simulink library "pathFollowingControllerExpStateMachine_cl"  (R2020a)
settings: Solver=VariableStepAuto  StartTime=0.0  StopTime=10.0  RelTol=1e-3
undefined symbols (not defined in the file or in its folder): env, FLIGHTCONTROLLER, fltCtrl, initializeBussesFromBlock, vhcl
libraries: simulink x6, filteredPIDController_ul x3, velocityAngle_ul x3, eulAng2RotMat_ul x2, stopwatch_ul x1, dspsigops x1, courseFollowExp_cl x1, ctrlAllocMatrixExp_cl x1, angleBtw2Vecs_ul x1, vrlib x1, alphaBeta_ul x1, gnd2TanRotation_ul x1
settings Model: Creator=jldanie5  LastModifiedBy=jcreed2
settings DataIOCC: ReturnWorkspaceOutputs=off
settings DebuggingCC: ArithmeticOperatorsInVariantConditions=warning
settings SFSimCC: CustomCodeUndefinedFunction=UseInterfaceOnly

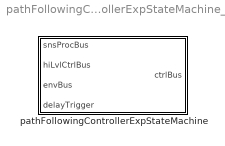
== system pathFollowingControllerExpStateMachine_cl ==
  pathFollowingControllerExpStateMachine : Subsystem  LoadFcn=initializeBussesFromBlock(gcb)  InitFcn=initializeBussesFromBlock(gcb)  StartFcn=initializeBussesFromBlock(gcb)  VariantControl=strcmpi(FLIGHTCONTROLLER,'pathFollowingControllerMantaBandLin')  mask{initPosForInitSStar=vhcl.initPosVecGnd.Value, fluidDensity=env.water.density.Value, pathCtrl=fltCtrl, aeroStruct=vhcl.struct('OCT.aeroSurf'), thrAttach=vhcl.rBridle_LE.Value, vhcl=vhcl}
      mask prompts: initPosForInitSStar "Initial Position"; fluidDensity "Fluid Density"; pathCtrl "Controller"; aeroStruct "Aerodynamic Structure"; thrAttach "Tether Attach Point"; vhcl "Vehicle"
      settings: MinAlgLoopOccurrences=on
      mask DialogControl Container3 Prompt: courseFollow Params
      mask DialogControl Container4 Prompt: setpointToOutput Params

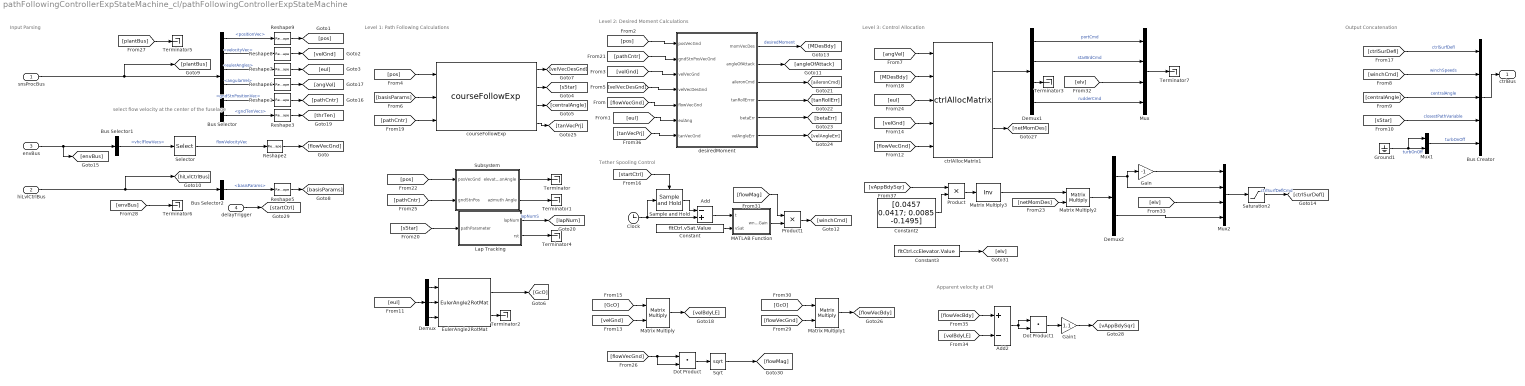
== system pathFollowingControllerExpStateMachine_cl/pathFollowingControllerExpStateMachine ==
  note: select flow velocity at the center of the fuselage
  note: Level 3: Control Allocation
  note: Output Concatenation
  note: Tether Spooling Control
  note: Level 2: Desired Moment Calculations
  note: Level 1: Path Following Calculations
  note: Input Parsing
  note: Apparent velocity at CM
  snsProcBus : Inport  OutDataTypeStr=Bus: sensorsProcessingBus
  hiLvlCtrlBus : Inport  Port=2  OutDataTypeStr=Bus: hiLvlCtrlBus
  envBus : Inport  Port=3  OutDataTypeStr=Bus: envBus
  delayTrigger : Inport  Port=4
  Add : Sum  Inputs=-+
  Add2 : Sum  Inputs=+-
  Bus Creator : BusCreator  Inputs=5  OutDataTypeStr=Bus: fltCtrlBus
      settings: InheritFromInputs=off
  Bus Selector : BusSelector  OutputSignals=positionVec,velocityVec,eulerAngles,angularVel,gndStnPositionVec,gndTenVecs
  Bus Selector1 : BusSelector  OutputSignals=vhclFlowVecs
  Bus Selector2 : BusSelector  OutputSignals=basisParams
  Clock : Clock
  Constant : Constant  Value=fltCtrl.vSat.Value
  Constant2 : Constant  Value=[0.0457 0.0417; 0.0085 -0.1495]
  Constant3 : Constant  Value=fltCtrl.ccElevator.Value
  Demux : Demux  Outputs=3
  Demux1 : Demux
  Demux2 : Demux  Outputs=2
  Dot Product : DotProduct  InputSameDT=on  OutDataTypeStr=Inherit: Inherit via internal rule
  Dot Product1 : DotProduct  InputSameDT=on  OutDataTypeStr=Inherit: Inherit via internal rule
  EulerAngle2RotMat : eulAng2RotMat_ul/EulerAngle2RotMat  SystemSampleTime=-1  Latency=0  AutoFrameSizeCalculation=off
  Gain : Gain  Gain=-1
  Gain1 : Gain  Gain=1.1
  Ground1 : Ground
  Lap Tracking : Subsystem
  MATLAB Function : MATLAB Function  TreatAsAtomicUnit=on
  Matrix Multiply : Product  Multiplication=Matrix(*)
  Matrix Multiply1 : Product  Multiplication=Matrix(*)
  Matrix Multiply2 : Product  Multiplication=Matrix(*)
  Matrix Multiply3 : Product  Inputs=/  Multiplication=Matrix(*)
  Mux : Mux
  Mux1 : Mux  Inputs=2
  Mux2 : Mux
  Product : Product
  Product1 : Product
  Reshape{1..3,5..9} (8 alike) : Reshape  OutputDimensionality=Column vector (2-D)
  Sample and Hold : dspsigops/Sample and Hold  trig=Rising edge  initCond=0  latchinput=off
  Saturation2 : Saturate  UpperLimit=pathCtrl.controlSigMax.upperLimit.Value  LowerLimit=pathCtrl.controlSigMax.lowerLimit.Value
  Selector : Selector  NumberOfDimensions=2  InputPortWidth=3  IndexOptions=Select all,Index vector (dialog)  Indices=[1 3],5  OutputSizes=1,1
  Sqrt : Sqrt  SaturateOnIntegerOverflow=on
  Subsystem : Subsystem
  Terminator{,1..7} (8 alike) : Terminator
  courseFollowExp : courseFollowExp_cl/courseFollowExp  SystemSampleTime=-1  Latency=0  AutoFrameSizeCalculation=off
  ctrlAllocMatrix1 : ctrlAllocMatrixExp_cl/ctrlAllocMatrix  aeroStruct=vhcl.struct('OCT.aeroSurf')  fluidDensity=fluidDensity
  desiredMoment : Subsystem
  ctrlBus : Outport  OutDataTypeStr=Bus: fltCtrlBus  VectorParamsAs1DForOutWhenUnconnected=off
  wires:
  Bus Selector/6 -> Reshape3/1  "<gndTenVecs>"
  Reshape3/1 -> [thrTen]
  courseFollowExp/1 -> [velVecDesGnd]
  snsProcBus/1 -> Bus Selector/1, [plantBus]
  Bus Selector/2 -> Reshape8/1  "<velocityVec>"
  Bus Selector/1 -> Reshape9/1  "<positionVec>"
  Bus Selector/3 -> Reshape7/1  "<eulerAngles>"
  [pos] -> courseFollowExp/1
  Bus Creator/1 -> ctrlBus/1
  [winchCmd] -> Bus Creator/2  "winchSpeeds"
  courseFollowExp/2 -> [sStar]
  hiLvlCtrlBus/1 -> [hiLvlCtrlBus], Bus Selector2/1
  [centralAngle] -> Bus Creator/3  "centralAngle"
  [sStar] -> Bus Creator/4  "closestPathVariable"
  courseFollowExp/3 -> [centralAngle]
  desiredMoment/1(momVecDes) -> [MDesBdy]  "desiredMoment"
  Bus Selector/4 -> Reshape6/1  "<angularVel>"
  [angVel] -> ctrlAllocMatrix1/1
  Demux1/3 -> Terminator3/1
  Demux1/1 -> Mux/1  "portCmd"
  Demux1/2 -> Mux/2  "starBrdCmd"
  ctrlAllocMatrix1/1 -> Demux1/1
  [ctrlSurDefl] -> Bus Creator/1  "ctrlSurfDefl"
  Bus Selector2/1 -> Reshape5/1  "<basisParams>"
  Reshape5/1 -> [basisParams]
  Saturation2/1 -> [ctrlSurDefl]  "ctrlSurfDeflCmd"
  Reshape2/1 -> [flowVecGnd]
  Reshape6/1 -> [angVel]
  Reshape7/1 -> [eul]
  Reshape8/1 -> [velGnd]
  Reshape9/1 -> [pos]
  Selector/1 -> Reshape2/1  "flowVelocityVec"
  envBus/1 -> [envBus], Bus Selector1/1
  Bus Selector1/1 -> Selector/1  "<vhclFlowVecs>"
  Reshape1/1 -> [pathCntr]
  Bus Selector/5 -> Reshape1/1  "<gndStnPositionVec>"
  [pathCntr] -> courseFollowExp/3
  [pos] -> desiredMoment/1(posVecGnd)
  [pathCntr] -> desiredMoment/2(gndStnPosVecGnd)
  [velGnd] -> desiredMoment/3(velVecGnd)
  [velVecDesGnd] -> desiredMoment/4(velVecDesGnd)
  [eul] -> desiredMoment/6(eulAng)
  [flowVecGnd] -> desiredMoment/5(flowVecGnd)
  [basisParams] -> courseFollowExp/2
  Demux1/4 -> Mux/4  "rudderCmd"
  Mux1/1 -> Bus Creator/5  "turbOnOff"
  [pos] -> Subsystem/1(posVecGnd)
  Subsystem/1(elevationAngle) -> Terminator/1
  Subsystem/2(azimuth Angle) -> Terminator1/1
  [elv] -> Mux/3
  desiredMoment/2(angleOfAttack) -> [angleOfAttack]
  [sStar] -> Lap Tracking/1(pathParameter)
  Lap Tracking/2(rst) -> Terminator4/1
  Lap Tracking/1(lapNum) -> [lapNum]  "lapNumS"
  [plantBus] -> Terminator5/1
  [envBus] -> Terminator6/1
  Constant/1 -> MATLAB Function/2(vSat)
  desiredMoment/3(aileronCmd) -> [aileronCmd]
  Mux/1 -> Terminator7/1
  desiredMoment/4(tanRollError) -> [tanRollErr]
  desiredMoment/5(betaErr) -> [betaErr]
  desiredMoment/6(velAngleErr) -> [velAngleErr]
  courseFollowExp/4 -> [tanVecPrj]
  [tanVecPrj] -> desiredMoment/7(tanVecGnd)
  [velGnd] -> ctrlAllocMatrix1/4
  [eul] -> ctrlAllocMatrix1/3
  [flowVecGnd] -> ctrlAllocMatrix1/5
  [MDesBdy] -> ctrlAllocMatrix1/2
  [pathCntr] -> Subsystem/2(gndStnPos)
  Ground1/1 -> Mux1/1, Mux1/2  "turbOnOff"
  [eul] -> Demux/1
  Demux/2 -> EulerAngle2RotMat/2
  Demux/1 -> EulerAngle2RotMat/1
  Demux/3 -> EulerAngle2RotMat/3
  EulerAngle2RotMat/2 -> Terminator2/1
  EulerAngle2RotMat/1 -> [GcO]
  [velGnd] -> Matrix Multiply/2
  [GcO] -> Matrix Multiply/1
  Matrix Multiply/1 -> [velBdyLE]
  Matrix Multiply1/1 -> [flowVecBdy]
  [GcO] -> Matrix Multiply1/1
  [flowVecGnd] -> Matrix Multiply1/2
  Constant2/1 -> Product/2
  Matrix Multiply2/1 -> Demux2/1
  Demux2/1 -> Mux2/2, Gain/1
  Gain/1 -> Mux2/1
  [elv] -> Mux2/3
  Demux2/2 -> Mux2/4
  Add2/1 -> Dot Product1/1, Dot Product1/2
  [flowVecBdy] -> Add2/1
  [velBdyLE] -> Add2/2
  Product/1 -> Matrix Multiply3/1
  Matrix Multiply3/1 -> Matrix Multiply2/1
  ctrlAllocMatrix1/2 -> [netMomDes]
  Dot Product1/1 -> Gain1/1
  [netMomDes] -> Matrix Multiply2/2
  [vAppBdySqr] -> Product/1
  Gain1/1 -> [vAppBdySqr]
  delayTrigger/1 -> [startCtrl]
  [startCtrl] -> Sample and Hold/Trigger
  Clock/1 -> Add/2, Sample and Hold/1
  Sample and Hold/1 -> Add/1
  Add/1 -> MATLAB Function/1(t)
  [flowVecGnd] -> Dot Product/2, Dot Product/1
  Dot Product/1 -> Sqrt/1
  Sqrt/1 -> [flowMag]
  MATLAB Function/1(wnchGain) -> Product1/2
  [flowMag] -> Product1/1
  Product1/1 -> [winchCmd]
  Constant3/1 -> [elv]
  Mux2/1 -> Saturation2/1

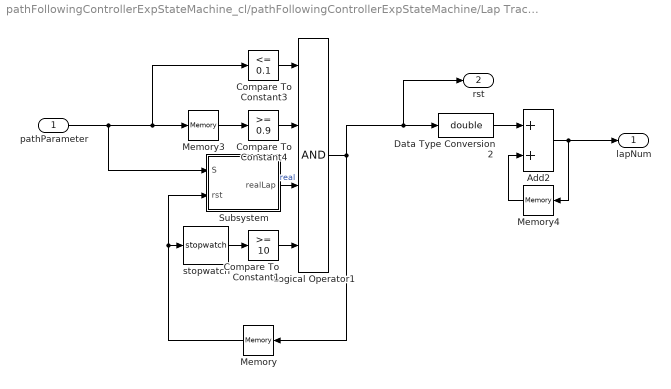
== system pathFollowingControllerExpStateMachine_cl/pathFollowingControllerExpStateMachine/Lap Tracking ==
  pathParameter : Inport
  Add2 : Sum
  Compare To Constant1 : simulink/Logic and Bit Operations/Compare To Constant  relop=>=  const=10  OutDataTypeStr=boolean
  Compare To Constant3 : simulink/Logic and Bit Operations/Compare To Constant  relop=<=  const=0.1  OutDataTypeStr=boolean
  Compare To Constant4 : simulink/Logic and Bit Operations/Compare To Constant  relop=>=  const=0.9  OutDataTypeStr=boolean
  Data Type Conversion2 : DataTypeConversion  OutDataTypeStr=double
  Logical Operator1 : Logic  Inputs=4  AllPortsSameDT=off  OutDataTypeStr=boolean
  Memory : Memory  InitialCondition=false
  Memory3 : Memory
  Memory4 : Memory
  Subsystem : Subsystem
  stopwatch : stopwatch_ul/stopwatch  SystemSampleTime=-1  Latency=0  AutoFrameSizeCalculation=off
  lapNum : Outport  VectorParamsAs1DForOutWhenUnconnected=off
  rst : Outport  Port=2  VectorParamsAs1DForOutWhenUnconnected=off
  wires:
  Compare To Constant3/1 -> Logical Operator1/1
  Memory3/1 -> Compare To Constant4/1
  Data Type Conversion2/1 -> Add2/1
  Logical Operator1/1 -> rst/1, Data Type Conversion2/1, Memory/1
  Memory4/1 -> Add2/2
  Add2/1 -> lapNum/1, Memory4/1
  Compare To Constant4/1 -> Logical Operator1/2
  pathParameter/1 -> Subsystem/1(S), Compare To Constant3/1, Memory3/1
  stopwatch/1 -> Compare To Constant1/1
  Memory/1 -> Subsystem/2(rst), stopwatch/1
  Compare To Constant1/1 -> Logical Operator1/4
  Subsystem/1(realLap) -> Logical Operator1/3  "real"

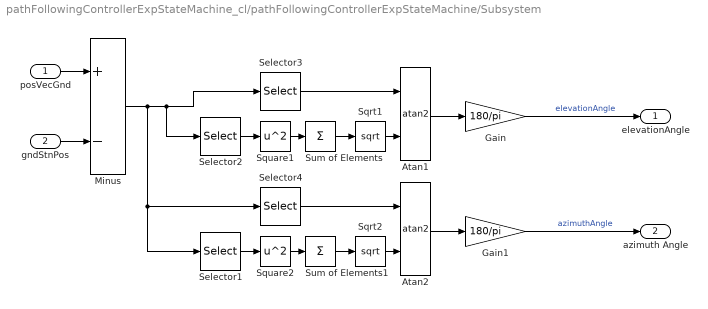
== system pathFollowingControllerExpStateMachine_cl/pathFollowingControllerExpStateMachine/Subsystem ==
  posVecGnd : Inport
  gndStnPos : Inport  Port=2
  Atan1 : Trigonometry  Operator=atan2
  Atan2 : Trigonometry  Operator=atan2
  Gain : Gain  Gain=180/pi
  Gain1 : Gain  Gain=180/pi
  Minus : Sum  Inputs=+-
  Selector1 : Selector  InputPortWidth=3  IndexOptions=Index vector (dialog)  Indices=1  OutputSizes=1
  Selector2 : Selector  InputPortWidth=3  IndexOptions=Index vector (dialog)  Indices=[1 2]  OutputSizes=1
  Selector3 : Selector  InputPortWidth=3  IndexOptions=Index vector (dialog)  Indices=3  OutputSizes=1
  Selector4 : Selector  InputPortWidth=3  IndexOptions=Index vector (dialog)  Indices=2  OutputSizes=1
  Sqrt1 : Sqrt  SaturateOnIntegerOverflow=on
  Sqrt2 : Sqrt  SaturateOnIntegerOverflow=on
  Square1 : Math  Operator=square  SignedPower=on  SaturateOnIntegerOverflow=on
  Square2 : Math  Operator=square  SignedPower=on  SaturateOnIntegerOverflow=on
  Sum of Elements : Sum  Inputs=+
  Sum of Elements1 : Sum  Inputs=+
  elevationAngle : Outport
  azimuth Angle : Outport  Port=2
  wires:
  Gain1/1 -> azimuth Angle/1  "azimuthAngle"
  Selector4/1 -> Atan2/1
  Sqrt2/1 -> Atan2/2
  Selector1/1 -> Square2/1
  Sum of Elements1/1 -> Sqrt2/1
  Square2/1 -> Sum of Elements1/1
  Atan2/1 -> Gain1/1
  Gain/1 -> elevationAngle/1  "elevationAngle"
  Selector2/1 -> Square1/1
  Atan1/1 -> Gain/1
  Sum of Elements/1 -> Sqrt1/1
  Selector3/1 -> Atan1/1
  Square1/1 -> Sum of Elements/1
  Sqrt1/1 -> Atan1/2
  posVecGnd/1 -> Minus/1
  gndStnPos/1 -> Minus/2
  Minus/1 -> Selector4/1, Selector1/1, Selector2/1, Selector3/1

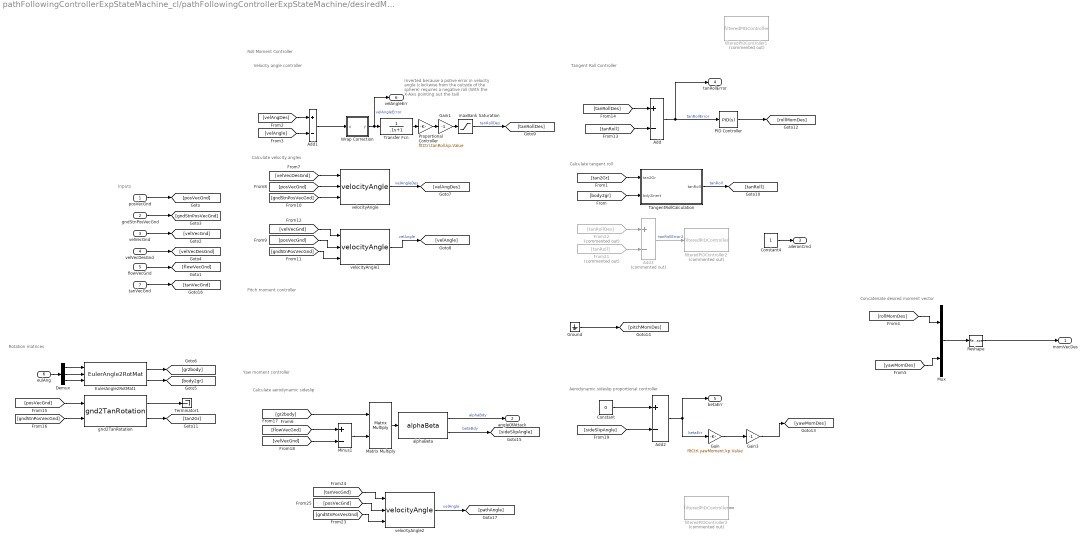
== system pathFollowingControllerExpStateMachine_cl/pathFollowingControllerExpStateMachine/desiredMoment ==
  note: Yaw moment controller
  note: Pitch moment controller
  note: Inverted because a potive error
      | in velocity angle (clockwise from the
      | outside of the sphere) requires a negative
      | roll (With the X-Axis pointing out the tail)
  note: Velocity angle controller
  note: Inputs
  note: Rotation matrices
  note: Calculate velocity angles
  note: Calculate tangent roll
  note: Tangent Roll Controller
  note: Concatenate desired moment vector
  note: Roll Moment Controller
  note: Aerodynamic sideslip proportional controller
  note: Calculate aerodynamic sideslip
  posVecGnd : Inport
  gndStnPosVecGnd : Inport  Port=2
  velVecGnd : Inport  Port=3
  velVecDesGnd : Inport  Port=4
  flowVecGnd : Inport  Port=5
  eulAng : Inport  Port=6
  tanVecGnd : Inport  Port=7
  Add : Sum  Inputs=+-
  Add1 : Sum  Inputs=+-
  Add2 : Sum  Inputs=+-
  Add3 : Sum  Commented=on  Inputs=+-
  Constant : Constant  Value=0
  Constant4 : Constant
  Demux : Demux  Outputs=3
  EulerAngle2RotMat1 : eulAng2RotMat_ul/EulerAngle2RotMat  SystemSampleTime=-1  Latency=0  AutoFrameSizeCalculation=off
  From21 : From  Commented=on  GotoTag=tanRoll
  From22 : From  Commented=on  GotoTag=tanRollDes
  Gain : Gain  Gain=fltCtrl.yawMoment.kp.Value
  Gain1 : Gain  Gain=-1
  Gain3 : Gain  Gain=-1
  Ground : Ground
  Matrix Multiply : Product  Multiplication=Matrix(*)
  Minus1 : Sum  Inputs=+-
  Mux : Mux  Inputs=2
  PID Controller : simulink/Continuous/PID Controller  Controller=PID  Form=Parallel  TimeDomain=Continuous-time  UseExternalTs=off  SampleTime=-1  IntegratorMethod=Forward Euler  FilterMethod=Forward Euler  ControllerParametersSource=internal  P=fltCtrl.rollMoment.kp.Value  I=0  D=fltCtrl.rollMoment.kd.Value  UseFilter=on  N=100  TunerSelectOption=Transfer Function Based (PID Tuner App)  InitialConditionSource=internal  InitialConditionForIntegrator=0  InitialConditionForFilter=0  DifferentiatorICPrevScaledInput=0  ExternalReset=none  TrackingMode=off  Kt=1  LimitOutput=off  UpperSaturationLimit=inf  LowerSaturationLimit=-inf  LinearizeAsGain=on  AntiWindupMode=none  Kb=1  POutMin=[]  POutMax=[]  IOutMin=[]  IOutMax=[]  DOutMin=[]  DOutMax=[]  NOutMin=[]  NOutMax=[]  SumOutMin=[]  SumOutMax=[]  SaturationOutMin=[]  SaturationOutMax=[]  PParamMin=[]  PParamMax=[]  IParamMin=[]  IParamMax=[]  DParamMin=[]  DParamMax=[]  NParamMin=[]  NParamMax=[]  KbParamMin=[]  KbParamMax=[]  KtParamMin=[]  KtParamMax=[]  KbOutMin=[]  KbOutMax=[]  KtOutMin=[]  KtOutMax=[]  IntegratorOutMin=[]  IntegratorOutMax=[]  FilterOutMin=[]  FilterOutMax=[]  SumI1OutMin=[]  SumI1OutMax=[]  SumI2OutMin=[]  SumI2OutMax=[]  SumI3OutMin=[]  SumI3OutMax=[]  SumI4OutMin=[]  SumI4OutMax=[]  SumDOutMin=[]  SumDOutMax=[]  DifferentiatorOutMin=[]  DifferentiatorOutMax=[]  FilterDiffOutCoefMin=[]  FilterDiffOutCoefMax=[]  ReciprocalOutMin=[]  ReciprocalOutMax=[]  SumDenOutMin=[]  SumDenOutMax=[]  SumNumOutMin=[]  SumNumOutMax=[]  DivideOutMin=[]  DivideOutMax=[]  UdiffTsProdOutMin=[]  UdiffTsProdOutMax=[]  NTsProdOutMin=[]  NTsProdOutMax=[]  UintegralTsProdOutMin=[]  UintegralTsProdOutMax=[]  UngainTsProdOutMin=[]  UngainTsProdOutMax=[]  IntegratorContinuousStateAttributes=''  IntegratorStateMustResolveToSignalObject=off  IntegratorRTWStateStorageClass=Auto  FilterContinuousStateAttributes=''  FilterStateMustResolveToSignalObject=off  FilterRTWStateStorageClass=Auto  ParallelPVariant=InternalParameters  IdealPVariant=Disabled  IVariant=InternalParameters  DVariant=InternalParameters  IntegratorVariant=Continuous  SatVariant=Disabled  AWVariant=Passthrough  PCopyVariant=Disabled  TRVariant=Disabled  FdbkBlocksVariant=Forward  IdealPFdbkVariant=Disabled  SatFdbkVariant=Disabled  DerivativeFilterVariant=ContFilter  NVariant=InternalParameters  NCopyVariant=Disabled  FilterICVariant=InternalICsFilter  IntegratorICVariant=InternalICs  ExternalResetVariant=Disabled  TRSumVariant=Passthrough  SumFdbkVariant=Disabled  SumVariant=Sum_PID  TsampFilterVariant=InternalTs  TsampNgainVariant=Passthrough  TsampIntegralVariant=Passthrough
  Proportional Controller : Gain  Gain=fltCtrl.tanRoll.kp.Value
  Reshape : Reshape  OutputDimensionality=Column vector (2-D)
  TangentRollCalculation : Subsystem
  Terminator1 : Terminator
  Transfer Fcn : TransferFcn  Denominator=[.1 1]
  Wrap Correction : Subsystem
  alphaBeta : alphaBeta_ul/alphaBeta  SystemSampleTime=-1  Latency=0  AutoFrameSizeCalculation=off
  filteredPIDController1 : filteredPIDController_ul/filteredPIDController  Commented=on  kp=pathCtrl.rollMoment.kp.Value  ki=0  kd=pathCtrl.rollMoment.kd.Value  Value=pathCtrl.rollMoment.tau.Value  externalReset=none
  filteredPIDController2 : filteredPIDController_ul/filteredPIDController  Commented=on  kp=fltCtrl.rollCtrl.kp.Value  ki=fltCtrl.rollCtrl.ki.Value  kd=fltCtrl.rollCtrl.kd.Value  Value=fltCtrl.rollCtrl.tau.Value  externalReset=none
  filteredPIDController3 : filteredPIDController_ul/filteredPIDController  Commented=on  kp=pathCtrl.yawMoment.kp.Value  ki=0  kd=pathCtrl.yawMoment.kd.Value  Value=pathCtrl.yawMoment.tau.Value  externalReset=none
  gnd2TanRotation : gnd2TanRotation_ul/gnd2TanRotation  SystemSampleTime=-1  Latency=0  AutoFrameSizeCalculation=off
  maxBank Saturation : Saturate  UpperLimit=pathCtrl.maxBank.upperLimit.Value  LowerLimit=pathCtrl.maxBank.lowerLimit.Value
  velocityAngle : velocityAngle_ul/velocityAngle  SystemSampleTime=-1  Latency=0  AutoFrameSizeCalculation=off
  velocityAngle1 : velocityAngle_ul/velocityAngle  SystemSampleTime=-1  Latency=0  AutoFrameSizeCalculation=off
  velocityAngle2 : velocityAngle_ul/velocityAngle  SystemSampleTime=-1  Latency=0  AutoFrameSizeCalculation=off
  momVecDes : Outport  VectorParamsAs1DForOutWhenUnconnected=off
  angleOfAttack : Outport  Port=2  VectorParamsAs1DForOutWhenUnconnected=off
  aileronCmd : Outport  Port=3  VectorParamsAs1DForOutWhenUnconnected=off
  tanRollError : Outport  Port=4
  betaErr : Outport  Port=5
  velAngleErr : Outport  Port=6
  wires:
  [yawMomDes] -> Mux/2
  gnd2TanRotation/1 -> Terminator1/1
  gnd2TanRotation/2 -> [tan2Gr]
  [gndStnPosVecGnd] -> gnd2TanRotation/2
  [posVecGnd] -> gnd2TanRotation/1
  [tanRollDes] -> Add/1
  [tanRoll] -> Add/2
  [velVecGnd] -> velocityAngle1/1
  [gndStnPosVecGnd] -> velocityAngle1/3
  [gndStnPosVecGnd] -> velocityAngle/3
  [posVecGnd] -> velocityAngle1/2
  [posVecGnd] -> velocityAngle/2
  [velVecDesGnd] -> velocityAngle/1
  [velAngle] -> Add1/2
  [velAngDes] -> Add1/1
  velocityAngle1/1 -> [velAngle]  "velAngle"
  velocityAngle/1 -> [velAngDes]  "velAngleDes"
  velVecDesGnd/1 -> [velVecDesGnd]
  gndStnPosVecGnd/1 -> [gndStnPosVecGnd]
  alphaBeta/1 -> angleOfAttack/1  "alphaBdy"
  Add2/1 -> Gain/1, betaErr/1  "betaErr"
  alphaBeta/2 -> [sideSlipAngle]  "betaBdy"
  Matrix Multiply/1 -> alphaBeta/1
  [gr2body] -> Matrix Multiply/1
  [body2gr] -> TangentRollCalculation/2(bdy2Inert)
  EulerAngle2RotMat1/1 -> [gr2body]
  EulerAngle2RotMat1/2 -> [body2gr]
  Demux/2 -> EulerAngle2RotMat1/2
  Demux/1 -> EulerAngle2RotMat1/1
  Demux/3 -> EulerAngle2RotMat1/3
  eulAng/1 -> Demux/1
  [flowVecGnd] -> Minus1/1
  [velVecGnd] -> Minus1/2
  Minus1/1 -> Matrix Multiply/2
  filteredPIDController3/1 -> ?
  TangentRollCalculation/1(tanRoll) -> [tanRoll]  "tanRoll"
  [tan2Gr] -> TangentRollCalculation/1(tan2Gr)
  flowVecGnd/1 -> [flowVecGnd]
  Add1/1 -> Wrap Correction/1(u)
  maxBank Saturation/1 -> [tanRollDes]  "tanRollDes"
  Gain1/1 -> maxBank Saturation/1
  Proportional Controller/1 -> Gain1/1
  Add/1 -> PID Controller/1, tanRollError/1  "tanRollError"
  velVecGnd/1 -> [velVecGnd]
  posVecGnd/1 -> [posVecGnd]
  Ground/1 -> [pitchMomDes]
  Transfer Fcn/1 -> Proportional Controller/1
  Add3/1 -> filteredPIDController2/1  "tanRollError2"
  From21/1 -> Add3/2
  From22/1 -> Add3/1
  tanVecGnd/1 -> [tanVecGnd]
  [gndStnPosVecGnd] -> velocityAngle2/3
  velocityAngle2/1 -> [pathAngle]  "velAngle"
  [tanVecGnd] -> velocityAngle2/1
  [posVecGnd] -> velocityAngle2/2
  Wrap Correction/1(y) -> velAngleErr/1, Transfer Fcn/1  "velAngleError"
  Mux/1 -> Reshape/1
  [rollMomDes] -> Mux/1
  Gain3/1 -> [yawMomDes]
  Constant4/1 -> aileronCmd/1
  Reshape/1 -> momVecDes/1
  [sideSlipAngle] -> Add2/2
  PID Controller/1 -> [rollMomDes]
  Gain/1 -> Gain3/1
  Constant/1 -> Add2/1

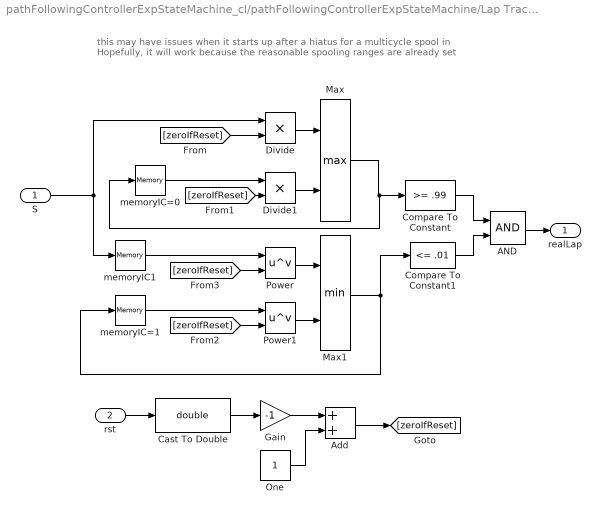
== system pathFollowingControllerExpStateMachine_cl/pathFollowingControllerExpStateMachine/Lap Tracking/Subsystem ==
  note: this may have issues when it starts up after a hiatus for a multicycle spool in
      | Hopefully, it will work because the reasonable spooling ranges are already set
  S : Inport
  rst : Inport  Port=2
  AND : Logic  AllPortsSameDT=off  OutDataTypeStr=boolean
  Add : Sum
  Cast To Double : DataTypeConversion  OutDataTypeStr=double
  Compare To Constant : simulink/Logic and Bit Operations/Compare To Constant  relop=>=  const=.99  OutDataTypeStr=boolean
  Compare To Constant1 : simulink/Logic and Bit Operations/Compare To Constant  relop=<=  const=.01  OutDataTypeStr=boolean
  Divide : Product  Inputs=**
  Divide1 : Product  Inputs=**
  Gain : Gain  Gain=-1
  Max : MinMax  Function=max  Inputs=2
  Max1 : MinMax  Inputs=2
  One : Constant  OutDataTypeStr=Inherit: Inherit via back propagation
  Power : Math  Operator=pow  SaturateOnIntegerOverflow=on
  Power1 : Math  Operator=pow  SaturateOnIntegerOverflow=on
  memoryIC1 : Memory  InitialCondition=1
  memoryIC=0 : Memory
  memoryIC=1 : Memory  InitialCondition=1
  realLap : Outport
  wires:
  Max1/1 -> Compare To Constant1/1, memoryIC=1/1
  rst/1 -> Cast To Double/1
  S/1 -> Divide/1, memoryIC1/1
  Gain/1 -> Add/1
  Add/1 -> [zeroIfReset]
  One/1 -> Add/2
  Divide/1 -> Max/1
  Max/1 -> memoryIC=0/1, Compare To Constant/1
  Power/1 -> Max1/1
  Power1/1 -> Max1/2
  Cast To Double/1 -> Gain/1
  Compare To Constant/1 -> AND/1
  Compare To Constant1/1 -> AND/2
  AND/1 -> realLap/1
  [zeroIfReset] -> Divide/2
  [zeroIfReset] -> Power/2
  [zeroIfReset] -> Divide1/2
  Divide1/1 -> Max/2
  memoryIC=0/1 -> Divide1/1
  [zeroIfReset] -> Power1/2
  memoryIC=1/1 -> Power1/1
  memoryIC1/1 -> Power/1

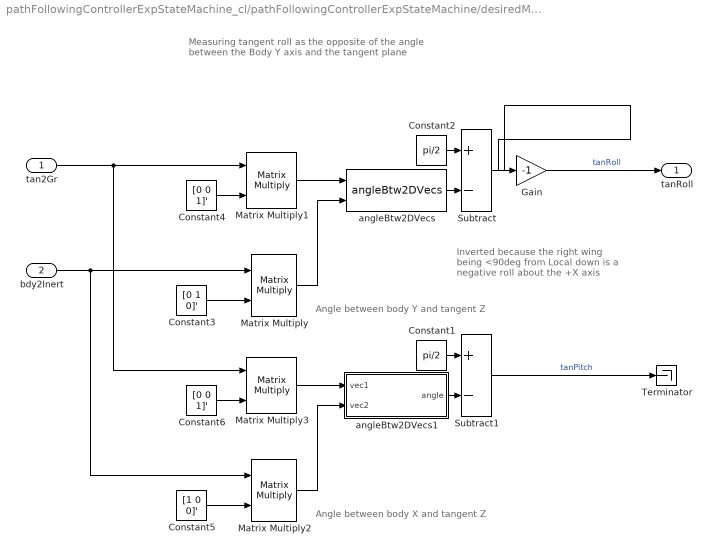
== system pathFollowingControllerExpStateMachine_cl/pathFollowingControllerExpStateMachine/desiredMoment/TangentRollCalculation ==
  note: Angle between body X and tangent Z
  note: Inverted because the right wing
      | being <90deg from Local down
      | is a negative roll about the +X axis
  note: Angle between body Y and tangent Z
  note: Measuring tangent roll as the opposite
      | of the angle between the Body Y axis
      | and the tangent plane
  tan2Gr : Inport
  bdy2Inert : Inport  Port=2
  Constant1 : Constant  Value=pi/2
  Constant2 : Constant  Value=pi/2
  Constant3 : Constant  Value=[0 1 0]'
  Constant4 : Constant  Value=[0 0 1]'
  Constant5 : Constant  Value=[1 0 0]'
  Constant6 : Constant  Value=[0 0 1]'
  Gain : Gain  Gain=-1
  Matrix Multiply{,1..3} (4 alike) : Product  Multiplication=Matrix(*)
  Subtract : Sum  Inputs=+-
  Subtract1 : Sum  Inputs=+-
  Terminator : Terminator
  angleBtw2DVecs : angleBtw2Vecs_ul/angleBtw2DVecs  SystemSampleTime=-1  Latency=0  AutoFrameSizeCalculation=off
  angleBtw2DVecs1 : Subsystem
  tanRoll : Outport  VectorParamsAs1DForOutWhenUnconnected=off
  wires:
  Constant5/1 -> Matrix Multiply2/2
  angleBtw2DVecs1/1(angle) -> Subtract1/2
  Constant1/1 -> Subtract1/1
  Matrix Multiply3/1 -> angleBtw2DVecs1/1(vec1)
  Constant6/1 -> Matrix Multiply3/2
  Matrix Multiply2/1 -> angleBtw2DVecs1/2(vec2)
  tan2Gr/1 -> Matrix Multiply1/1, Matrix Multiply3/1
  Subtract1/1 -> Terminator/1  "tanPitch"
  bdy2Inert/1 -> Matrix Multiply/1, Matrix Multiply2/1
  Gain/1 -> tanRoll/1  "tanRoll"
  Matrix Multiply/1 -> angleBtw2DVecs/2
  Constant4/1 -> Matrix Multiply1/2
  Matrix Multiply1/1 -> angleBtw2DVecs/1
  Constant2/1 -> Subtract/1
  angleBtw2DVecs/1 -> Subtract/2
  Constant3/1 -> Matrix Multiply/2
  Subtract/1 -> Gain/1

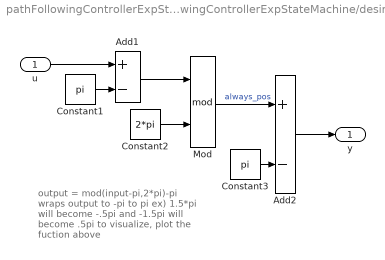
== system pathFollowingControllerExpStateMachine_cl/pathFollowingControllerExpStateMachine/desiredMoment/Wrap Correction ==
  note: output = mod(input-pi,2*pi)-pi
      | wraps output to -pi to pi
      |
      | ex) 1.5*pi will become -.5pi
      | 	and -1.5pi will become .5pi
      |
      | to visualize, plot the fuction above
  u : Inport
  Add1 : Sum  Inputs=+-
  Add2 : Sum  Inputs=+-
  Constant1 : Constant  Value=pi
  Constant2 : Constant  Value=2*pi
  Constant3 : Constant  Value=pi
  Mod : Math  Operator=mod  SignedPower=on  SaturateOnIntegerOverflow=on
  y : Outport  VectorParamsAs1DForOutWhenUnconnected=off
  wires:
  Add2/1 -> y/1
  Constant3/1 -> Add2/2
  Mod/1 -> Add2/1  "always_pos"
  Constant2/1 -> Mod/2
  Add1/1 -> Mod/1
  Constant1/1 -> Add1/2
  u/1 -> Add1/1

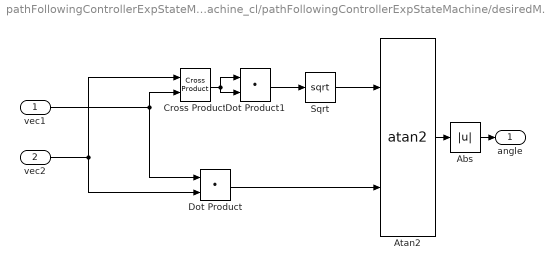
== system pathFollowingControllerExpStateMachine_cl/pathFollowingControllerExpStateMachine/desiredMoment/TangentRollCalculation/angleBtw2DVecs1 ==
  vec1 : Inport
  vec2 : Inport  Port=2
  Abs : Abs
  Atan2 : Trigonometry  Operator=atan2
  Cross Product : vrlib/Utilities/Cross Product
      settings: SourceProductBaseCode=VR
  Dot Product : DotProduct  InputSameDT=on  OutDataTypeStr=Inherit: Inherit via internal rule
  Dot Product1 : DotProduct  InputSameDT=on  OutDataTypeStr=Inherit: Inherit via internal rule
  Sqrt : Sqrt  SaturateOnIntegerOverflow=on
  angle : Outport  VectorParamsAs1DForOutWhenUnconnected=off
  wires:
  Sqrt/1 -> Atan2/1
  Dot Product1/1 -> Sqrt/1
  Abs/1 -> angle/1
  Dot Product/1 -> Atan2/2
  Cross Product/1 -> Dot Product1/2, Dot Product1/1
  vec2/1 -> Dot Product/2, Cross Product/1
  vec1/1 -> Cross Product/2, Dot Product/1
  Atan2/1 -> Abs/1

== matlab function pathFollowingControllerExpStateMachine_cl/pathFollowingControllerExpStateMachine/MATLAB Function ==
  data: t input; wnchGain output; vSat input
function wnchGain   = fcn(t,vSat)
wnchGain = 0;
if t< 15 || t>150
    wnchGain = 0;
else
    wnchGain = .001*(t-15)^2;
end

if wnchGain >= vSat
    wnchGain = vSat;
end
